simulink model "aTestModelOLD"  (R2015a)
settings: Solver=ode45  StartTime=0.0  StopTime=10  RelTol=1e-6
values from neighbouring files (symbols this model uses):
  B_f = 6.08e-3    (= 0.00608)    [aTestComparison.m]    (also in aTestComparisonOLD.m)
  B_w = 17.03e-6    (= 1.703e-05)    [aTestComparison.m]    (also in aTestComparisonOLD.m)
  g = 9.82    [aTestComparison.m]    (also in aTestComparisonOLD.m)
  J_f = (2.8e-3)    (= 0.0028)    [aTestComparison.m]    (also in aTestComparisonOLD.m)
  J_w = 0.601e-3    (= 0.000601)    [aTestComparison.m]    (also in aTestComparisonOLD.m)
  l_f = 0.076    [aTestComparison.m]    (also in aTestComparisonOLD.m)
  l_w = 0.093    [aTestComparison.m]    (also in aTestComparisonOLD.m)
  m_f = 0.354    [aTestComparison.m]    (also in aTestComparisonOLD.m)
  m_w = 0.222    [aTestComparison.m]    (also in aTestComparisonOLD.m)
settings Model: CovSFcnEnable=off  Creator=USUARIO  LastModifiedBy=vniel
settings DataIOCC: LimitDataPoints=off
settings DebuggingCC: SolverPrmCheckMsg=warning

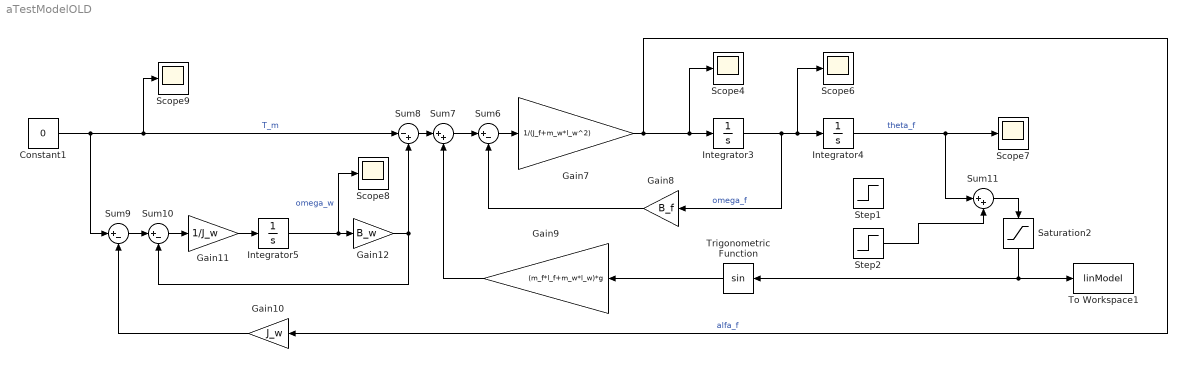
== system aTestModelOLD ==
  Constant1 : Constant  Value=0
  Gain10 : Gain  Gain=J_w
  Gain11 : Gain  Gain=1/J_w
  Gain12 : Gain  Gain=B_w
  Gain7 : Gain  Gain=1/(J_f+m_w*l_w^2)
  Gain8 : Gain  Gain=B_f
  Gain9 : Gain  Gain=(m_f*l_f+m_w*l_w)*g
  Integrator3 : Integrator
  Integrator4 : Integrator
  Integrator5 : Integrator
  Saturation2 : Saturate  UpperLimit=0.85  LowerLimit=-0.72
  Scope{4,6..9} (5 alike) : Scope
      Scope4 settings: YMin=-10  YMax=10  SaveName=ScopeData2
      Scope6 settings: YMin=-10  YMax=10  SaveName=ScopeData4
      Scope7 settings: TimeRange=2  YMin=0  YMax=14000  SaveName=StepResponseData1
      Scope8 settings: YMin=-10  YMax=10  SaveName=ScopeData6
      Scope9 settings: YMin=-10  YMax=10  SaveName=ScopeData7
  Step1 : Step  Time=0.0001  Before=-0.001  After=0  SampleTime=0
  Step2 : Step  Time=0  After=-0.1475  SampleTime=0
  Sum10 : Sum  Inputs=|+-
  Sum11 : Sum  Inputs=|++
  Sum6 : Sum  Inputs=|+-
  Sum7 : Sum  Inputs=|++
  Sum8 : Sum  Inputs=|-+
  Sum9 : Sum  Inputs=|+-
  To Workspace1 : ToWorkspace  VariableName=linModel  SaveFormat=Timeseries  SampleTime=-1
  Trigonometric Function : Trigonometry
  wires:
  Gain7/1 -> Gain10/1, Scope4/1, Integrator3/1  "alfa_f"
  Integrator3/1 -> Gain8/1, Scope6/1, Integrator4/1  "omega_f"
  Sum6/1 -> Gain7/1
  Sum7/1 -> Sum6/1
  Gain8/1 -> Sum6/2
  Gain9/1 -> Sum7/2
  Sum8/1 -> Sum7/1
  Sum10/1 -> Gain11/1
  Gain11/1 -> Integrator5/1
  Gain10/1 -> Sum9/2
  Sum9/1 -> Sum10/1
  Integrator5/1 -> Scope8/1, Gain12/1  "omega_w"
  Gain12/1 -> Sum10/2, Sum8/2
  Constant1/1 -> Sum9/1, Scope9/1, Sum8/1  "T_m"
  Integrator4/1 -> Scope7/1, Sum11/1  "theta_f"
  Sum11/1 -> Saturation2/1
  Saturation2/1 -> Trigonometric Function/1, To Workspace1/1
  Trigonometric Function/1 -> Gain9/1
  Step2/1 -> Sum11/2
